simulink model "HevP2TransmissionController"  (R2020a)
settings: Solver=FixedStepDiscrete  StartTime=0.0  StopTime=inf  FixedStep=0.01  RelTol=1e-3  EnableMultiTasking=on
model workspace (MAT data in the model file):
  Dn_Shft_Spd = [3  7  11  15  19; 3  7  11  15  19; 10  17  26  35  49; 10  17  26  35  49]
  Gear_Dn_bpt = [2 3 4 5 6]
  Gear_Up_bpt = [1 2 3 4 5]
  Pdl_Pos_Dn_bpt = [0 0.6 0.9 1]
  Pdl_Pos_Up_bpt = [0 0.25 0.9 1]
  Up_Shft_Spd = [5  9  13  17  21; 5  9  13  17  21; 12  19  28  37  51; 12  19  28  37  51]
settings Model: ModifiedByFormat=The MathWorks, Inc.  Creator=The MathWorks, Inc.  LastModifiedBy=The MathWorks, Inc.
settings SolverCC: AutoInsertRateTranBlk=on
settings DataIOCC: SaveOutput=off  SaveTime=off  ReturnWorkspaceOutputs=off
settings DebuggingCC: ArithmeticOperatorsInVariantConditions=warning
settings SFSimCC: SimUseLocalCustomCode=off  CustomCodeUndefinedFunction=UseInterfaceOnly
settings RTWCC: RTWUseLocalCustomCode=off
settings CodeAppCC: StateflowObjectComments=on

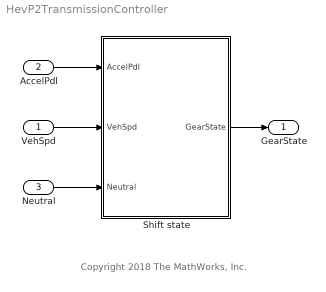
== system HevP2TransmissionController ==
  note: Copyright 2018 The MathWorks, Inc.
  VehSpd : Inport  OutDataTypeStr=double  PortDimensions=1
  AccelPdl : Inport  Port=2  OutDataTypeStr=double  PortDimensions=1
  Neutral : Inport  Port=3
  Shift state : Subsystem
  GearState : Outport  VectorParamsAs1DForOutWhenUnconnected=off
  wires:
  AccelPdl/1 -> Shift state/1(AccelPdl)
  VehSpd/1 -> Shift state/2(VehSpd)
  Neutral/1 -> Shift state/3(Neutral)
  Shift state/1(GearState) -> GearState/1

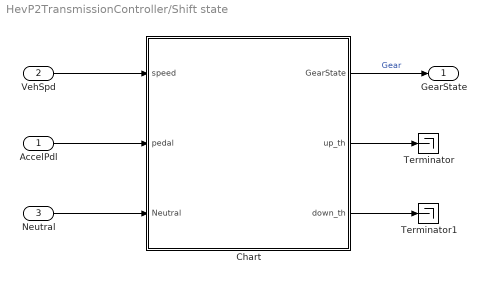
== system HevP2TransmissionController/Shift state ==
  AccelPdl : Inport
  VehSpd : Inport  Port=2
  Neutral : Inport  Port=3
  Chart : Stateflow chart  TreatAsAtomicUnit=on
  Terminator : Terminator
  Terminator1 : Terminator
  GearState : Outport  VectorParamsAs1DForOutWhenUnconnected=off
  wires:
  AccelPdl/1 -> Chart/2(pedal)
  Chart/1(GearState) -> GearState/1  "Gear"
  Chart/3(down_th) -> Terminator1/1
  Chart/2(up_th) -> Terminator/1
  Neutral/1 -> Chart/3(Neutral)
  VehSpd/1 -> Chart/1(speed)

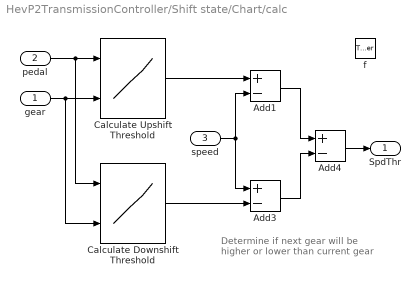
== system HevP2TransmissionController/Shift state/Chart/calc ==
  note: Determine if next gear will be
      | higher or lower than current gear
  gear : Inport
  pedal : Inport  Port=2
  speed : Inport  Port=3
  f : TriggerPort  TriggerType=function-call  VariantControl=Variant  StatesWhenEnabling=reset
      settings: CopyFcn=Stateflow.SLINSF.SimulinkMan.removeBlockPreDeleteFcn  PreDeleteFcn=Stateflow.SLINSF.SimulinkMan.unsafePredeleteFcn
  Add1 : Sum  Inputs=+-
  Add3 : Sum  Inputs=+-
  Add4 : Sum  Inputs=+-
  Calculate Upshift Threshold : Lookup_n-D  BreakpointsForDimension1=Pdl_Pos_Up_bpt  BreakpointsForDimension2=Gear_Up_bpt  Table=Up_Shft_Spd  ExtrapMethod=Clip  UseLastTableValue=on  InternalRulePriority=Speed  RndMeth=Simplest  InputSameDT=on
  Calculate Downshift Threshold : Lookup_n-D  BreakpointsForDimension1=Pdl_Pos_Dn_bpt  BreakpointsForDimension2=Gear_Dn_bpt  Table=Dn_Shft_Spd  ExtrapMethod=Clip  UseLastTableValue=on  InternalRulePriority=Speed  RndMeth=Simplest  InputSameDT=on
  SpdThr : Outport  VectorParamsAs1DForOutWhenUnconnected=off
  wires:
  pedal/1 -> Calculate Downshift Threshold/1, Calculate Upshift Threshold/1
  gear/1 -> Calculate Downshift Threshold/2, Calculate Upshift Threshold/2
  Calculate Downshift Threshold/1 -> Add3/2
  Calculate Upshift Threshold/1 -> Add1/1
  speed/1 -> Add1/2, Add3/1
  Add1/1 -> Add4/1
  Add3/1 -> Add4/2
  Add4/1 -> SpdThr/1

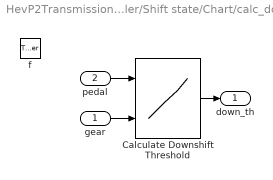
== system HevP2TransmissionController/Shift state/Chart/calc_down ==
  gear : Inport
  pedal : Inport  Port=2
  f : TriggerPort  TriggerType=function-call  VariantControl=Variant  StatesWhenEnabling=reset
      settings: CopyFcn=Stateflow.SLINSF.SimulinkMan.removeBlockPreDeleteFcn  PreDeleteFcn=Stateflow.SLINSF.SimulinkMan.unsafePredeleteFcn
  Calculate Downshift Threshold : Lookup_n-D  BreakpointsForDimension1=Pdl_Pos_Dn_bpt  BreakpointsForDimension2=Gear_Dn_bpt  Table=Dn_Shft_Spd  ExtrapMethod=Clip  UseLastTableValue=on  InternalRulePriority=Speed  RndMeth=Simplest  InputSameDT=on
  down_th : Outport  VectorParamsAs1DForOutWhenUnconnected=off
  wires:
  Calculate Downshift Threshold/1 -> down_th/1
  gear/1 -> Calculate Downshift Threshold/2
  pedal/1 -> Calculate Downshift Threshold/1

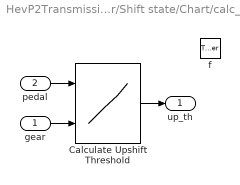
== system HevP2TransmissionController/Shift state/Chart/calc_up ==
  gear : Inport
  pedal : Inport  Port=2
  f : TriggerPort  TriggerType=function-call  VariantControl=Variant  StatesWhenEnabling=reset
      settings: CopyFcn=Stateflow.SLINSF.SimulinkMan.removeBlockPreDeleteFcn  PreDeleteFcn=Stateflow.SLINSF.SimulinkMan.unsafePredeleteFcn
  Calculate Upshift Threshold : Lookup_n-D  BreakpointsForDimension1=Pdl_Pos_Up_bpt  BreakpointsForDimension2=Gear_Up_bpt  Table=Up_Shft_Spd  ExtrapMethod=Clip  UseLastTableValue=on  InternalRulePriority=Speed  RndMeth=Simplest  InputSameDT=on
  up_th : Outport  VectorParamsAs1DForOutWhenUnconnected=off
  wires:
  Calculate Upshift Threshold/1 -> up_th/1
  pedal/1 -> Calculate Upshift Threshold/1
  gear/1 -> Calculate Upshift Threshold/2

== stateflow chart HevP2TransmissionController/Shift state/Chart ==
  settings: sampleTime=0.01  enableNonTerminalStates=1
  state GearState [parallel]
    settings: executionOrder=1
    state Neutral
      en:
      GearState = 0;
    state G1
      en:
      GearState = 1;
    state G2
      en:
      GearState = 2;
      du:
      [SpdThr] = calc(2,pedal,speed);
    state G3
      en:
      GearState = 3;
      du:
      [SpdThr] = calc(3,pedal,speed);
    state G6
      en:
      GearState = 6;
    state G5
      en:GearState=5;
      du:[SpdThr]=calc(5,pedal,speed);
    state G4
      en:
      GearState = 4;
      du:
      [SpdThr] = calc(4,pedal,speed);
    (default) -> G1
    Neutral -> G1 : [~Neutral]
    G1 -> G2 [order 1] : Up
    G2 -> G3 [order 1] : Up
    G1 -> Neutral [order 2] : [Neutral]
    G2 -> G1 [order 2] : Down
    G3 -> G2 [order 2] : Down
    G3 -> G4 [order 1] : Up
    G4 -> G3 [order 2] : Down
    G5 -> G6 [order 1] : Up
    G4 -> G5 [order 1] : Up
    G5 -> G4 [order 2] : Down
    G6 -> G5 : Down
  state SelectionState [parallel]
    du:[up_th]=calc_up(GearState,pedal);
    du:[down_th]=calc_down(GearState,pedal);
    settings: executionOrder=2
    state SteadyState
      en:
      clutchControl = 0;
    state preDownShifting
    state preUpShifting
    state UpShifting
      en:
      GearState = GearState + 0.5;
    state DownShifting
      en:
      GearState = GearState - 0.5;
    (default) -> SteadyState
    SteadyState -> (junction 62) [order 1] : [speed < down_th && ...
        | GearState >1]
    SteadyState -> (junction 128) [order 2] : [speed > up_th &&...
        | GearState <= 5 && ...
        | floor(GearState) == GearState]
    (junction 62) -> preDownShifting
    (junction 128) -> preUpShifting
    (junction 168) -> SteadyState
    (junction 23) -> SteadyState
    (junction 161) -> SteadyState
    preDownShifting -> (junction 168) [order 2] : [speed >= down_th]
    preUpShifting -> (junction 161) [order 2] : [speed <= up_th]
    preUpShifting -> UpShifting [order 1] : after(0.5,sec)
        | [speed>up_th]
    preDownShifting -> DownShifting [order 1] : after(0.5, sec)
        | [speed < down_th - 2]
    DownShifting -> (junction 23) : {GearState.Down;}
    UpShifting -> (junction 23) : {GearState.Up;}
  state up_th = calc_up(gear,pedal) [function]
  state down_th = calc_down(gear,pedal) [function]
  state SpdThr = calc(gear,pedal,speed) [function]
  data: gear function_input; pedal function_input; up_th function_output; gear function_input; pedal function_input; down_th function_output; gear function_input; pedal function_input; SpdThr function_output; speed function_input; GearState output double =1; speed input; pedal input; up_th output double; down_th output double; clutchControl local double; SpdThr local double; Neutral input
  events: Up local EITHER_EDGE_EVENT; Down local EITHER_EDGE_EVENT
